simulink model "soc_WLAN_fpga"  (R2024b)
settings: Solver=FixedStepDiscrete  StartTime=0.0  StopTime=stopTime  RelTol=1e-3
PreLoadFcn:
  | addpath(fullfile(matlabroot,'toolbox','whdl','whdlexamples','whdlexamples'));
InitFcn:
  | addpath(fullfile(matlabroot,'toolbox','whdl','whdlexamples','whdlexamples'));
model workspace (MAT data in the model file):
  socvcb : containers.Map (value not decoded)
undefined symbols (not defined in the file): Add, bitRatePerOfdmSym, chanBW, coe, cpLen, dataUpsampleFactor, DelayValMaxNsdMinusLastPilotSc, DescramblerInitialSeed, designMultirateFIR, fftLen, filterLatency, filterUpsampleFactor, Fs, Hd, HT_MFMCS0, HT_MFMCS1, HT_MFMCS2, HT_MFMCS3, HT_MFMCS4, HT_MFMCS5, HT_MFMCS6, HT_MFMCS7, HTUnUsedScInd, inputSamplingRate, interp_coeff, maxPilotRefCounterVale, maxPilotsRef, maxPilotsRefNonHT, Ncol_HT, Ncol_NonHT, noDataSubCarriers, Non_HTMCS0, Non_HTMCS1, Non_HTMCS2, Non_HTMCS3, Non_HTMCS4, Non_HTMCS5, Non_HTMCS6, Non_HTMCS7, Nrow_HT, Nrow_NonHT, numDSC_HT, numDSC_HT_vhtSigB, numDSC_NonHT, numDscHT, numDscNonHT, numOfBitsPerOFDMSym, numOfDataBitsPerOFDMSym, numPilots, numScHT, numSCS_HT, numSCS_NonHT, pnSeq, QAM, rxDownsampleFactor, secondPIdx_HT, secondPIdx_NonHT, Shift, VHTMCS0, VHTMCS1 ... (+7)
libraries: hdlsllib x267, simulink x210, dspsigops x22, whdlutilities x10, whdlmod x9, dsphdlfiltering2 x5, dsphdlmathfun2 x4, whdledac x3, hwlogicconnlib x2, commhdlcrc x2, dsphdlsigops2 x2
(part 2 of 14)

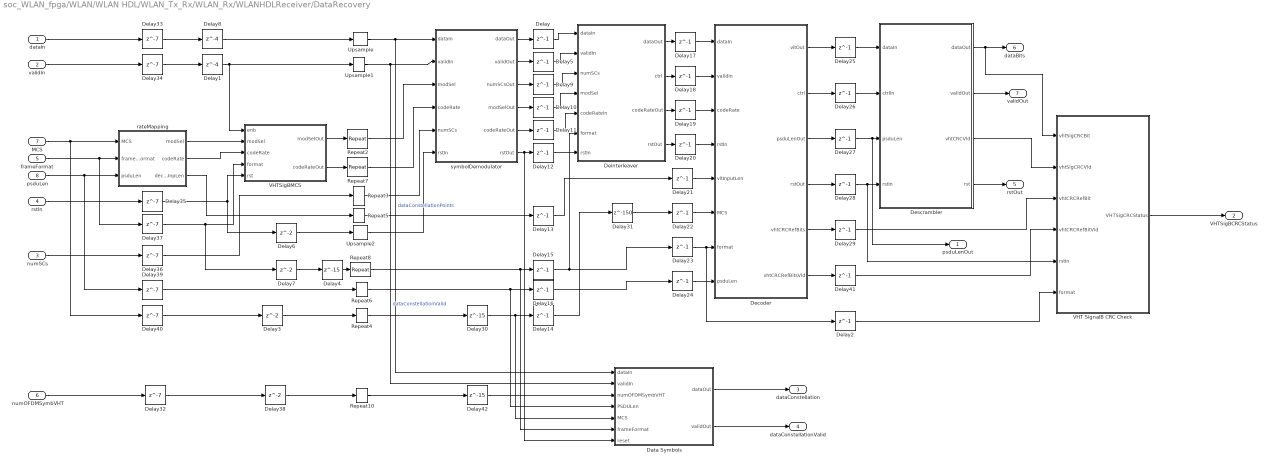
== system soc_WLAN_fpga/WLAN/WLAN HDL/WLAN_Tx_Rx/WLAN_Rx/WLANHDLReceiver/DataRecovery ==
  dataIn : Inport
  validIn : Inport  Port=2
  numSCs : Inport  Port=3
  rstIn : Inport  Port=4
  frameFormat : Inport  Port=5
  numOFDMSymbVHT : Inport  Port=6
  MCS : Inport  Port=7
  psduLen : Inport  Port=8
  Data Symbols : Subsystem
  Decoder : Subsystem
  Deinterleaver : Subsystem
  Delay{,2,5,9..29,41} (25 alike) : Delay  DelayLength=1
  Delay1 : Delay  DelayLength=4
  Delay{3,6..7,38} (4 alike) : Delay
  Delay30 : Delay  DelayLength=15
  Delay31 : Delay  DelayLength=150
  Delay{32..37,39..40} (8 alike) : Delay  DelayLength=7
  Delay4 : Delay  DelayLength=15
  Delay42 : Delay  DelayLength=15
  Delay8 : Delay  DelayLength=4
  Descrambler : Subsystem
  Repeat{2..8,10} (8 alike) : dspsigops/Repeat  FactorSource=Dialog parameter  N=dataUpsampleFactor  Nmax=16  RateOptions=Allow multirate processing  ic=0  mode=Unused parameter value
  Upsample : dspsigops/Upsample  FactorSource=Dialog parameter  N=dataUpsampleFactor  Nmax=16  phase=0  RateOptions=Allow multirate processing  ic=0  mode=Unused parameter value
  Upsample1 : dspsigops/Upsample  FactorSource=Dialog parameter  N=dataUpsampleFactor  Nmax=16  phase=0  RateOptions=Allow multirate processing  ic=0  mode=Unused parameter value
  Upsample2 : dspsigops/Upsample  FactorSource=Dialog parameter  N=dataUpsampleFactor  Nmax=16  phase=0  RateOptions=Allow multirate processing  ic=0  mode=Unused parameter value
  VHT SignalB CRC Check : Subsystem
  VHTSigBMCS : Subsystem
  rateMapping : Subsystem
  symbolDemodulator : Subsystem
  psduLenOut : Outport
  VHTSigBCRCStatus : Outport  Port=2
  dataConstellation : Outport  Port=3
  dataConstellationValid : Outport  Port=4
  rstOut : Outport  Port=5
  dataBits : Outport  Port=6
  validOut : Outport  Port=7
  wires:
  Descrambler/2(validOut) -> validOut/1
  Descrambler/1(dataOut) -> VHT SignalB CRC Check/1(vhtSigCRCBit), dataBits/1
  Upsample1/1 -> symbolDemodulator/2(validIn), Data Symbols/2(validIn)  "dataConstellationValid"
  Upsample/1 -> symbolDemodulator/1(dataIn), Data Symbols/1(dataIn)  "dataConstellationPoints"
  Delay28/1 -> VHT SignalB CRC Check/5(rstIn), Descrambler/4(rstIn)
  Delay26/1 -> Descrambler/2(ctrlIn)
  Delay25/1 -> Descrambler/1(dataIn)
  Delay24/1 -> Decoder/8(psduLen)
  Delay23/1 -> Delay2/1, Decoder/7(format)
  Delay22/1 -> Decoder/6(MCS)
  Delay21/1 -> Decoder/5(vitInputLen)
  Delay20/1 -> Decoder/4(rstIn)
  Delay19/1 -> Decoder/3(codeRate)
  Delay18/1 -> Decoder/2(validIn)
  Delay17/1 -> Decoder/1(dataIn)
  Delay16/1 -> Delay24/1
  Delay15/1 -> Deinterleaver/6(format), Delay23/1
  Delay14/1 -> Delay31/1
  Delay13/1 -> Delay21/1
  Delay12/1 -> Deinterleaver/7(rstIn)
  Delay11/1 -> Deinterleaver/5(codeRateIn)
  Delay10/1 -> Deinterleaver/4(modSel)
  Delay9/1 -> Deinterleaver/3(numSCs)
  Delay5/1 -> Deinterleaver/2(validIn)
  Delay/1 -> Deinterleaver/1(dataIn)
  Decoder/3(psduLenOut) -> Delay27/1
  Decoder/5(vhtCRCRefBits) -> Delay29/1
  symbolDemodulator/6(rstOut) -> Data Symbols/7(reset), Delay12/1
  rateMapping/3(decoderInpLen) -> Repeat5/1
  rateMapping/2(codeRate) -> VHTSigBMCS/3(codeRate)
  rateMapping/1(modSel) -> VHTSigBMCS/2(modSel)
  symbolDemodulator/5(codeRateOut) -> Delay11/1
  Deinterleaver/3(codeRateOut) -> Delay19/1
  Repeat7/1 -> symbolDemodulator/4(codeRate)
  VHTSigBMCS/1(modSelOut) -> Repeat2/1
  Delay7/1 -> Delay4/1
  frameFormat/1 -> Delay37/1, rateMapping/2(frameFormat)
  Delay6/1 -> Upsample2/1
  Decoder/4(rstOut) -> Delay28/1
  Deinterleaver/4(rstOut) -> Delay20/1
  Delay4/1 -> Repeat8/1
  Delay1/1 -> VHTSigBMCS/1(enb), Upsample1/1
  validIn/1 -> Delay34/1
  Delay8/1 -> Upsample/1
  Repeat4/1 -> Delay30/1
  MCS/1 -> Delay40/1, rateMapping/1(MCS)
  VHTSigBMCS/2(codeRateOut) -> Repeat7/1
  Repeat8/1 -> Data Symbols/6(frameFormat), Delay15/1
  Repeat6/1 -> Delay16/1, Data Symbols/4(PSDULen)
  Repeat5/1 -> Delay13/1
  Upsample2/1 -> symbolDemodulator/6(rstIn)
  Repeat3/1 -> symbolDemodulator/5(numSCs)
  Repeat2/1 -> symbolDemodulator/3(modSel)
  rstIn/1 -> Delay35/1
  symbolDemodulator/4(modSelOut) -> Delay10/1
  psduLen/1 -> Delay39/1, rateMapping/3(psduLen)
  Deinterleaver/2(ctrl) -> Delay18/1
  Deinterleaver/1(dataOut) -> Delay17/1
  Decoder/2(ctrl) -> Delay26/1
  Decoder/1(vitOut) -> Delay25/1
  numSCs/1 -> Delay36/1
  symbolDemodulator/2(validOut) -> Delay5/1
  symbolDemodulator/1(dataOut) -> Delay/1
  symbolDemodulator/3(numSCsOut) -> Delay9/1
  dataIn/1 -> Delay33/1
  Delay33/1 -> Delay8/1
  Delay34/1 -> Delay1/1
  Delay35/1 -> VHTSigBMCS/5(rst), Delay6/1
  Delay36/1 -> Repeat3/1
  Delay37/1 -> VHTSigBMCS/4(format), Delay7/1
  Delay39/1 -> Repeat6/1
  Delay40/1 -> Delay3/1
  Decoder/6(vhtCRCRefBitsVld) -> Delay41/1
  Descrambler/3(vhtCRCVld) -> VHT SignalB CRC Check/2(vhtSigCRCVld)
  Delay29/1 -> VHT SignalB CRC Check/3(vhtCRCRefBit)
  VHT SignalB CRC Check/1(VHTSigCRCStatus) -> VHTSigBCRCStatus/1
  Delay27/1 -> psduLenOut/1, Descrambler/3(psduLen)
  Data Symbols/2(validOut) -> dataConstellationValid/1
  Data Symbols/1(dataOut) -> dataConstellation/1
  Delay41/1 -> VHT SignalB CRC Check/4(vhtCRCRefBitVld)
  Delay2/1 -> VHT SignalB CRC Check/6(format)
  Delay3/1 -> Repeat4/1
  Delay30/1 -> Delay14/1, Data Symbols/5(MCS)
  Delay31/1 -> Delay22/1
  Delay32/1 -> Delay38/1
  Repeat10/1 -> Delay42/1
  Delay38/1 -> Repeat10/1
  numOFDMSymbVHT/1 -> Delay32/1
  Delay42/1 -> Data Symbols/3(numOFDMSymbVHT)
  Descrambler/4(rst) -> rstOut/1

== system soc_WLAN_fpga/WLAN/WLAN HDL/WLAN_Tx_Rx/WLAN_Rx/WLANHDLReceiver/FrameFormatController ==
  note: Appriopriate delays to match detected frame format arrival
  note: Choose L-Data from symbol 6
  NonHTDataIn : Inport
  NonHTValid : Inport  Port=2
  numSymb : Inport  Port=3
  NonHTRst : Inport  Port=4
  formatDetected : Inport  Port=5
  HTDataIn : Inport  Port=6
  HTValid : Inport  Port=7
  HTRst : Inport  Port=8
  Compare To Constant : simulink/Logic and Bit Operations/Compare To Constant  relop=>=  const=5  OutDataTypeStr=boolean
  Constant : Constant  Value=numDscHT  OutDataTypeStr=fixdt(0,16,0)  SampleTime=-1
  Constant1 : Constant  Value=numDscNonHT  OutDataTypeStr=fixdt(0,16,0)  SampleTime=-1
  Delay : Delay  DelayLength=388+64+160+64
  Delay10 : Delay  DelayLength=87+32+8*fftLen
  Delay11 : Delay  DelayLength=388+160+64+64
  Delay3 : Delay  DelayLength=87+32
  Delay4 : Delay  DelayLength=87+32
  Delay8 : Delay  DelayLength=388+64+160+64
  Delay9 : Delay  DelayLength=388+160+64+64
  Logical Operator : Logic  AllPortsSameDT=off  OutDataTypeStr=boolean
  Switch1 : Switch  Criteria=u2 > Threshold  SaturateOnIntegerOverflow=off  InputSameDT=off  OutDataTypeStr=Inherit: Same as first input
  Switch3 : Switch  Criteria=u2 > Threshold  SaturateOnIntegerOverflow=off  InputSameDT=off
  Switch4 : Switch  Criteria=u2 > Threshold  SaturateOnIntegerOverflow=off  InputSameDT=off
  Switch5 : Switch  Criteria=u2 > Threshold  SaturateOnIntegerOverflow=off  InputSameDT=off
  dataOut : Outport
  validOut : Outport  Port=2
  numSCs : Outport  Port=3
  rstOut : Outport  Port=4
  wires:
  Switch5/1 -> rstOut/1
  Switch1/1 -> dataOut/1
  Delay8/1 -> Logical Operator/1
  Constant/1 -> Switch4/1
  Compare To Constant/1 -> Logical Operator/2
  Constant1/1 -> Switch4/3
  Delay4/1 -> Switch1/1
  Delay/1 -> Compare To Constant/1
  Delay9/1 -> Switch1/3
  Switch4/1 -> numSCs/1
  Logical Operator/1 -> Switch3/3
  Delay3/1 -> Switch3/1
  Delay11/1 -> Switch5/3
  Delay10/1 -> Switch5/1
  numSymb/1 -> Delay/1
  HTRst/1 -> Delay10/1
  Switch3/1 -> validOut/1
  HTValid/1 -> Delay3/1
  HTDataIn/1 -> Delay4/1
  NonHTDataIn/1 -> Delay9/1
  NonHTValid/1 -> Delay8/1
  NonHTRst/1 -> Delay11/1
  formatDetected/1 -> Switch4/2, Switch5/2, Switch1/2, Switch3/2

== system soc_WLAN_fpga/WLAN/WLAN HDL/WLAN_Tx_Rx/WLAN_Rx/WLANHDLReceiver/FrameFormatDetectionAndSignalRecovery ==
  dataIn : Inport
  validIn : Inport  Port=2
  symbNum : Inport  Port=3
  rstIn : Inport  Port=4
  CRCCheckAndBitInterpretation : Subsystem
  Data Type Conversion : DataTypeConversion  OutDataTypeStr=fixdt(1,16,14)  SaturateOnIntegerOverflow=off  RndMeth=Floor
  Delay : Delay  DelayLength=18
  FormatIdentification : Subsystem
      settings: PortSchema="{\"entries\":[{\"content\":{\"sides\":[{\"content\":{\"connectorIds\":[\"In1\",\"In2\",\"In3\",\"In4\"]},\"type\":\"ConnectorPlacement.EquallySpacedRectSide\",\"uuid\":\"3028114e-cab1-417f-bebe-6d6476787930\"},{\"content\":{\"connectorIds\":[],\"side\":\"RIGHT\"},\"type\":\"ConnectorPlacement.EquallySpacedRectSide\",\"uuid\":\"6d8234fc-94fb-4772-a32f-944b1f5aeeb4\"},{\"content\":{\"connectorIds\":[\"Out2\",\"In5\"],\"side\":\"TOP\"},\"type\":\"ConnectorPlacement.EquallySpacedRectSide\",\"uuid\":\"0ff67b69-6efc-48c5-b813-d09036213c24\"},{\"content\":{\"connectorIds\":[\"Out1\"],\"side\":\"BOTTOM\"},\"type\":\"ConnectorPlacement.EquallySpacedRectSide\",\"uuid\":\"c34dfd74-148e-4ad2-9a51-cfec2f6e9138\"}]},\"type\":\"ConnectorPlacement.EquallySpacedConnector\",\"uuid\":\"49430930-ff4f-4485-8b33-823117f3dfd7\"}],\"packageUris\":[\"http://schema.mathworks.com/mf0/Connector/R2020b\"],\"version\":\"1.0\"}"
  Sample Control Bus Selector : whdlutilities/Sample Control Bus Selector  OutputSignals=start,end,valid
  SignalBitRecovery : Subsystem
  SignalFieldController : Subsystem
      settings: PortSchema="{\"entries\":[{\"content\":{\"sides\":[{\"content\":{\"connectorIds\":[\"In1\",\"In2\",\"In3\",\"In4\",\"In5\",\"In6\"]},\"type\":\"ConnectorPlacement.EquallySpacedRectSide\",\"uuid\":\"148ceb8f-1186-445b-b3f6-f8d5d753c1bf\"},{\"content\":{\"connectorIds\":[\"Out1\",\"Out2\",\"Out3\",\"Out4\"],\"side\":\"RIGHT\"},\"type\":\"ConnectorPlacement.EquallySpacedRectSide\",\"uuid\":\"6dacdfa0-ad7e-48bf-93e0-eecd8ec6f6a0\"},{\"content\":{\"connectorIds\":[],\"side\":\"TOP\"},\"type\":\"ConnectorPlacement.EquallySpacedRectSide\",\"uuid\":\"eaeaab77-8bbe-4397-bc6e-e6aaca64b8f0\"},{\"content\":{\"connectorIds\":[\"In7\"],\"side\":\"BOTTOM\"},\"type\":\"ConnectorPlacement.EquallySpacedRectSide\",\"uuid\":\"580f9177-349a-4b9d-9319-c70de4e7be3b\"}]},\"type\":\"ConnectorPlacement.EquallySpacedConnector\",\"uuid\":\"773ad17b-09fa-48bb-b0c0-63eaf23152dd\"}],\"packageUris\":[\"http://schema.mathworks.com/mf0/Connector/R2020b\"],\"version\":\"1.0\"}"
  Terminator10 : Terminator
  Terminator9 : Terminator
  averageSigFieldsFor40MHz : Subsystem
  storingSignalFields : Subsystem
      settings: PortSchema="{\"entries\":[{\"content\":{\"sides\":[{\"content\":{\"connectorIds\":[\"In1\",\"In2\",\"In3\",\"In4\"]},\"type\":\"ConnectorPlacement.EquallySpacedRectSide\",\"uuid\":\"994a7f9b-6ab5-43b4-a8d7-53561a33412d\"},{\"content\":{\"connectorIds\":[\"Out1\",\"Out2\"],\"side\":\"RIGHT\"},\"type\":\"ConnectorPlacement.EquallySpacedRectSide\",\"uuid\":\"f9668c3e-3593-48e7-8bc9-4614bf79b57c\"},{\"content\":{\"connectorIds\":[\"In5\"],\"side\":\"TOP\"},\"type\":\"ConnectorPlacement.EquallySpacedRectSide\",\"uuid\":\"29666b31-aec6-4c8c-a4b7-b4d610cf5f51\"}]},\"type\":\"ConnectorPlacement.EquallySpacedConnector\",\"uuid\":\"339975a6-4895-4382-8eec-20ecff8c26e4\"}],\"packageUris\":[\"http://schema.mathworks.com/mf0/Connector/R2020b\"],\"version\":\"1.0\"}"
  decodedMCS : Outport
  CRCCheck : Outport  Port=2
  frameFormat : Outport  Port=3
  PSDULength : Outport  Port=4
  HTCRCStatus : Outport  Port=5
  headerConstellation : Outport  Port=6
  numOFDMSymbVHT : Outport  Port=7
  wires:
  symbNum/1 -> FormatIdentification/3(symbCount), storingSignalFields/4(symbCount), SignalFieldController/5(symbNum)
  Sample Control Bus Selector/3 -> CRCCheckAndBitInterpretation/2(<valid>)  "<valid>"
  Sample Control Bus Selector/2 -> Terminator10/1  "<end>"
  SignalBitRecovery/2(ctrlOut) -> Sample Control Bus Selector/1
  Sample Control Bus Selector/1 -> Terminator9/1  "<start>"
  FormatIdentification/2(frameFormat) -> CRCCheckAndBitInterpretation/3(formatDetected), frameFormat/1, SignalFieldController/7(formatDetected)
  FormatIdentification/1(formatDetected) -> storingSignalFields/5(formatDetected)
  SignalFieldController/3(modSel) -> SignalBitRecovery/3(modSel)
  SignalFieldController/2(dataSCValid) -> SignalBitRecovery/2(dataSCValid)
  SignalFieldController/1(dataOut) -> SignalBitRecovery/1(dataIn)
  storingSignalFields/2(validOut) -> [HTSigSymbValid]
  [HTSigSymbValid] -> SignalFieldController/4(validOut)
  storingSignalFields/1(rd_dout) -> [HTSigSymbData]
  [HTSigSymbData] -> SignalFieldController/3(rd_dout)
  SignalBitRecovery/1(signBit) -> CRCCheckAndBitInterpretation/1(bit)
  rstIn/1 -> storingSignalFields/1(rst), FormatIdentification/4(rst), SignalFieldController/6(rst), SignalBitRecovery/4(rst), Delay/1, averageSigFieldsFor40MHz/3(rst)
  CRCCheckAndBitInterpretation/4(MCS) -> FormatIdentification/5(MCS), decodedMCS/1
  CRCCheckAndBitInterpretation/1(failCheck) -> CRCCheck/1
  CRCCheckAndBitInterpretation/2(PSDULen) -> PSDULength/1
  SignalBitRecovery/3(headerConstellation) -> headerConstellation/1
  CRCCheckAndBitInterpretation/3(HTCRCStatus) -> HTCRCStatus/1
  Data Type Conversion/1 -> storingSignalFields/2(dataIn), FormatIdentification/1(dataIn), SignalFieldController/1(dataIn)
  SignalFieldController/4(numSCS) -> SignalBitRecovery/5(numSCS)
  averageSigFieldsFor40MHz/2(Out2) -> SignalFieldController/2(validIn), storingSignalFields/3(validIn), FormatIdentification/2(validIn)
  dataIn/1 -> averageSigFieldsFor40MHz/1(In1)
  validIn/1 -> averageSigFieldsFor40MHz/2(In2)
  averageSigFieldsFor40MHz/1(Out1) -> Data Type Conversion/1
  Delay/1 -> CRCCheckAndBitInterpretation/4(rst)
  CRCCheckAndBitInterpretation/5(numOFDMSymbVHT) -> numOFDMSymbVHT/1

== system soc_WLAN_fpga/WLAN/WLAN HDL/WLAN_Tx_Rx/WLAN_Rx/WLANHDLReceiver/HT_VHTCPEEstAndCorrection ==
  dataIn : Inport
  validIn : Inport  Port=2
  vhtSigB : Inport  Port=3
  formatDetected : Inport  Port=4
  rstIn : Inport  Port=5
  CPECorrector : Subsystem
  CPEEstimator : Subsystem
  Data Type Conversion : DataTypeConversion  OutDataTypeStr=fixdt(1,16,10)  SaturateOnIntegerOverflow=off  RndMeth=Floor
  Data Type Conversion1 : DataTypeConversion  OutDataTypeStr=fixdt(1,16,14)  SaturateOnIntegerOverflow=off  RndMeth=Floor
  Delay{,1,3,9} (4 alike) : Delay
  Delay10 : Delay  DelayLength=3
  Delay11 : Delay  DelayLength=3
  Delay{12..23} (12 alike) : Delay  DelayLength=1  InitialCondition=0  UseCircularBuffer=on
  Delay2 : Delay  DelayLength=3
  Delay4 : Delay  DelayLength=fftLen
  Delay5 : Delay  DelayLength=fftLen
  Delay6 : Delay  DelayLength=fftLen
  Delay7 : Delay  DelayLength=1.5*(fftLen)
  Delay8 : Delay  DelayLength=94+56
  Logical Operator1 : Logic  AllPortsSameDT=off  OutDataTypeStr=boolean
  Logical Operator2 : Logic  Operator=NOT  AllPortsSameDT=off  OutDataTypeStr=boolean
  Logical Operator3 : Logic  Operator=OR  AllPortsSameDT=off  OutDataTypeStr=boolean
  PilotSubCarrierSelector : Subsystem
  PolarityGenerator : Subsystem
  dataOut : Outport
  validOut : Outport  Port=2
  rstOut : Outport  Port=3
  wires:
  Delay10/1 -> Data Type Conversion1/1
  Delay11/1 -> validOut/1
  Delay8/1 -> Delay2/1
  PilotSubCarrierSelector/3(SymbStart) -> PolarityGenerator/1(enb)
  PolarityGenerator/2(vhtSigB) -> CPEEstimator/5(vhtSigB)
  PilotSubCarrierSelector/2(SymbEndInd) -> Delay/1
  Logical Operator3/1 -> Delay16/1, PilotSubCarrierSelector/1(validIn)  "sampleIn"
  Delay/1 -> CPEEstimator/3(SymbolEndInd)
  Logical Operator2/1 -> Logical Operator1/2
  Delay9/1 -> Delay5/1
  Delay3/1 -> CPEEstimator/2(pilotScValid)
  Logical Operator1/1 -> Delay9/1  "sampleIn"
  Delay1/1 -> Data Type Conversion/1, CPEEstimator/1(dataOut)
  PolarityGenerator/1(polarity) -> CPEEstimator/4(polarity)
  PilotSubCarrierSelector/1(pilotScValidOut) -> Delay3/1, Logical Operator2/1  "sampleOut"
  CPECorrector/1(dataOut) -> Delay10/1
  validIn/1 -> Logical Operator3/1  "sampleIn"
  CPECorrector/2(validOut) -> Delay11/1
  Delay2/1 -> rstOut/1
  Data Type Conversion1/1 -> dataOut/1
  CPEEstimator/1(x) -> CPECorrector/3(estimate)
  formatDetected/1 -> Delay7/1
  Delay12/1 -> CPECorrector/1(dataIn)
  Delay13/1 -> CPECorrector/2(validIn)
  Delay14/1 -> Delay8/1
  Data Type Conversion/1 -> Delay4/1
  Delay6/1 -> Delay23/1
  Delay7/1 -> Delay17/1
  vhtSigB/1 -> Delay18/1, Logical Operator3/2
  dataIn/1 -> Delay15/1
  rstIn/1 -> Delay19/1, PilotSubCarrierSelector/2(rst)
  Delay5/1 -> Delay22/1
  Delay4/1 -> Delay21/1
  Delay15/1 -> Delay1/1
  Delay16/1 -> Logical Operator1/1
  Delay17/1 -> PolarityGenerator/2(formatDetected)
  Delay18/1 -> PolarityGenerator/3(VHTSigB)
  Delay19/1 -> Delay20/1, PolarityGenerator/4(rst)
  Delay20/1 -> Delay6/1, CPEEstimator/6(rst)
  Delay21/1 -> Delay12/1
  Delay22/1 -> Delay13/1
  Delay23/1 -> Delay14/1

== system soc_WLAN_fpga/WLAN/WLAN HDL/WLAN_Tx_Rx/WLAN_Rx/WLANHDLReceiver/HT_VHTChannelEstAndEqualize ==
  note: Delay by 1.4 times OFDM symbol length to match frame format detected
  note: HT/VHT scaling factor
  dataIn : Inport
  validIn : Inport  Port=2
  symbNum : Inport  Port=3
  symbRst : Inport  Port=4
  rstIn : Inport  Port=5
  formatIn : Inport  Port=6
  ChannelEqualizer : Subsystem
  ChannelEstimator : Subsystem
  Delay : Delay  DelayLength=80+32
  Delay15 : Delay  DelayLength=80+32
  Delay16 : Delay  DelayLength=80+32
  Delay{3..5,22..23} (5 alike) : Delay  DelayLength=14  InputProcessing=Columns as channels (frame based)
  Delay24 : Delay  DelayLength=94  InputProcessing=Columns as channels (frame based)
  Delay6 : Delay  DelayLength=94  InputProcessing=Columns as channels (frame based)
  Gain : Gain  Gain=fi(sqrt(numScHT),0,16,8)  OutDataTypeStr=fixdt(1,16,13)
  HTScSelector : Subsystem
  ValidController : Subsystem
  dataOut : Outport
  validOut : Outport  Port=2
  vhtSigBVld : Outport  Port=3
  formatOut : Outport  Port=4
  rstOut : Outport  Port=5
  wires:
  ChannelEstimator/3(chanEstLen) -> ChannelEqualizer/5(chanEstLen)
  Delay4/1 -> ChannelEqualizer/2(validIn)
  ChannelEstimator/1(HT_VHTchanEst) -> ChannelEqualizer/3(chanEst)
  HTScSelector/1(chanEstValid) -> Delay4/1, ChannelEstimator/2(validIn)
  Delay3/1 -> ChannelEqualizer/1(dataIn)
  Delay5/1 -> Delay6/1, ChannelEqualizer/7(symbNum)
  ChannelEstimator/2(HT_VHTchanEstValid) -> ChannelEqualizer/4(chanEstVal)
  ChannelEqualizer/2(validOut) -> Delay15/1  "sampleIn"
  ChannelEqualizer/1(dataOut) -> Delay16/1
  Delay6/1 -> Delay/1
  formatIn/1 -> ValidController/2(formatDetected), formatOut/1
  Delay/1 -> ValidController/1(symbNum)
  Delay15/1 -> ValidController/3(validIn)
  Delay22/1 -> ChannelEqualizer/6(syncStart)
  Delay23/1 -> Delay24/1
  dataIn/1 -> Gain/1
  ValidController/2(vhtSigB) -> vhtSigBVld/1
  Delay16/1 -> dataOut/1
  ValidController/1(validOut) -> validOut/1
  Delay24/1 -> rstOut/1
  validIn/1 -> HTScSelector/1(validIn)
  symbRst/1 -> HTScSelector/2(symbRst)
  Gain/1 -> ChannelEstimator/1(dataIn), Delay3/1
  rstIn/1 -> Delay23/1, Delay22/1, ChannelEstimator/3(syncStart), HTScSelector/3(rst)
  symbNum/1 -> Delay5/1, ChannelEstimator/4(symbNum)

== system soc_WLAN_fpga/WLAN/WLAN HDL/WLAN_Tx_Rx/WLAN_Rx/WLANHDLReceiver/NonHTCPEEstAndCorrection ==
  dataIn : Inport
  sampleIn : Inport  Port=2
  symbNum : Inport  Port=3
  rstIn : Inport  Port=4
  CPECorrector : Subsystem
  CPEEstimator : Subsystem
  DataSubCarrierSelector : Subsystem
  Delay{,3..4,7,9,11..25} (20 alike) : Delay  DelayLength=1  InitialCondition=0  UseCircularBuffer=on
  Delay1 : Delay  DelayLength=37
  Delay10 : Delay  DelayLength=fftLen
  Delay2 : Delay  DelayLength=37
  Delay5 : Delay  DelayLength=fftLen  InputProcessing=Columns as channels (frame based)
  Delay6 : Delay  DelayLength=fftLen  InputProcessing=Columns as channels (frame based)
  Delay8 : Delay  DelayLength=fftLen  InputProcessing=Columns as channels (frame based)
  PilotSubCarrierSelector : Subsystem
  PolarityGenerator : Subsystem
  dataOut : Outport
  validOut : Outport  Port=2
  symbNumOut : Outport  Port=3
  rstOut : Outport  Port=4
  wires:
  CPECorrector/2(validOut) -> validOut/1
  Delay8/1 -> Delay11/1
  CPECorrector/1(dataOut) -> dataOut/1
  Delay10/1 -> Delay9/1
  Delay5/1 -> Delay12/1
  PolarityGenerator/1(polarity) -> CPEEstimator/4(polarity)
  PilotSubCarrierSelector/3(SymbStart) -> PolarityGenerator/1(enb)
  CPEEstimator/1(x) -> CPECorrector/3(estimate)
  Delay6/1 -> Delay13/1
  DataSubCarrierSelector/1(dataScValidOut) -> Delay6/1  "sampleIn"
  PilotSubCarrierSelector/2(SymbEndInd) -> Delay17/1
  PilotSubCarrierSelector/1(pilotScValidOut) -> Delay16/1  "sampleOut"
  Delay1/1 -> rstOut/1
  Delay2/1 -> symbNumOut/1
  Delay/1 -> CPECorrector/1(dataIn)
  Delay3/1 -> CPECorrector/2(validIn)
  Delay4/1 -> Delay1/1
  Delay7/1 -> Delay2/1
  Delay9/1 -> Delay4/1
  Delay11/1 -> Delay7/1
  Delay12/1 -> Delay/1
  Delay13/1 -> Delay3/1
  Delay14/1 -> Delay8/1
  Delay15/1 -> CPEEstimator/5(rst), Delay10/1
  Delay16/1 -> CPEEstimator/2(pilotScValid)
  Delay17/1 -> CPEEstimator/3(SymbolEndInd)
  Delay18/1 -> CPEEstimator/1(dataOut)
  Delay20/1 -> Delay5/1
  sampleIn/1 -> Delay24/1, PilotSubCarrierSelector/1(EqValidIn)
  dataIn/1 -> Delay23/1, Delay25/1
  rstIn/1 -> Delay19/1, Delay22/1, PilotSubCarrierSelector/2(rst)
  symbNum/1 -> Delay21/1
  Delay19/1 -> Delay15/1
  Delay21/1 -> Delay14/1
  Delay22/1 -> DataSubCarrierSelector/2(rst), PolarityGenerator/2(rstIn)
  Delay23/1 -> Delay18/1
  Delay24/1 -> DataSubCarrierSelector/1(EqValidIn)
  Delay25/1 -> Delay20/1

== system soc_WLAN_fpga/WLAN/WLAN HDL/WLAN_Tx_Rx/WLAN_Rx/WLANHDLReceiver/NonHTChannelEstAndEqualize ==
  note: Non-HT scaling factor
  note: Select Non-HT frame format used subcarriers
  dataIn : Inport
  validIn : Inport  Port=2
  symbNum : Inport  Port=3
  symbRst : Inport  Port=4
  rstIn : Inport  Port=5
  ChannelEqualizer : Subsystem
  ChannelEstimator : Subsystem
  Delay{,1..2,8,14} (5 alike) : Delay
  Delay{10..13} (4 alike) : Delay  DelayLength=1
  Delay{3..5,7} (4 alike) : Delay  DelayLength=14  InputProcessing=Columns as channels (frame based)
  Delay6 : Delay  DelayLength=92  InputProcessing=Columns as channels (frame based)
  Delay9 : Delay  DelayLength=92  InputProcessing=Columns as channels (frame based)
  Gain : Gain  Gain=fi(sqrt(numSCS_NonHT),0,16,8)  OutDataTypeStr=fixdt(1,16,13)
  NonHTScSelector : Subsystem
  dataOut : Outport
  validOut : Outport  Port=2
  symbNumOut : Outport  Port=3
  rstOut : Outport  Port=4
  wires:
  Delay3/1 -> ChannelEqualizer/1(dataIn)
  Delay5/1 -> ChannelEqualizer/6(symbNum), Delay6/1
  Delay10/1 -> Delay3/1, ChannelEstimator/1(dataIn)
  Delay13/1 -> ChannelEstimator/4(syncStart), Delay7/1
  Delay9/1 -> rstOut/1
  Delay1/1 -> NonHTScSelector/1(validIn)
  Delay/1 -> Gain/1
  Delay11/1 -> ChannelEstimator/2(validIn), Delay4/1
  dataIn/1 -> Delay/1
  ChannelEstimator/2(chanEstValid) -> ChannelEqualizer/4(chanEstVal)
  Delay12/1 -> Delay5/1, ChannelEstimator/3(symbNum)
  ChannelEqualizer/2(validOut) -> validOut/1
  ChannelEqualizer/1(dataOut) -> dataOut/1
  symbNum/1 -> Delay2/1
  ChannelEstimator/3(chanEstLen) -> ChannelEqualizer/5(chanEstLen)
  rstIn/1 -> Delay8/1
  Delay6/1 -> symbNumOut/1
  Delay4/1 -> ChannelEqualizer/2(validIn)
  validIn/1 -> Delay1/1
  ChannelEstimator/1(chanEst) -> ChannelEqualizer/3(chanEst)
  NonHTScSelector/1(chanEstValid) -> Delay11/1
  Delay7/1 -> ChannelEqualizer/7(rst), Delay9/1
  symbRst/1 -> Delay14/1
  Delay14/1 -> NonHTScSelector/2(symbRst)
  Gain/1 -> Delay10/1
  Delay2/1 -> Delay12/1
  Delay8/1 -> Delay13/1, NonHTScSelector/3(rst)

== system soc_WLAN_fpga/WLAN/WLAN HDL/WLAN_Tx_Rx/WLAN_Rx/WLANHDLReceiver/OFDMDemodulation ==
  dataIn : Inport
  validIn : Inport  Port=2
  rstIn : Inport  Port=3
  Data Type Conversion : DataTypeConversion  OutDataTypeStr=fixdt(1,16,14)  SaturateOnIntegerOverflow=off  RndMeth=Floor
  Delay : Delay  DelayLength=278
  Delay{1..6} (6 alike) : Delay  DelayLength=1
  Delay7 : Delay
  Delay8 : Delay
  Delay9 : Delay
  Logical Operator : Logic  AllPortsSameDT=off  OutDataTypeStr=boolean
  Logical Operator1 : Logic  Operator=NOT  AllPortsSameDT=off  OutDataTypeStr=boolean
  OFDM Demodulator : whdlmod/OFDM Demodulator  OFDMParamsSource=Input port  MaxFFTLength=maxFFTLen  FFTLength=64  CPLength=16  NumLGsC=6  NumRGsC=5  CPFraction=off  CPFractionSource=Property  CPFractionValue=0.75  removeDCSubcarriers=off  enableResetInputPort=on  Normalize=on  RoundingMethod=Floor  SimulateUsing=Code generation
  OFDMDemodParamsCalculator : MATLAB Function  TreatAsAtomicUnit=on
  Symbol Counter : Subsystem
  Terminator4 : Terminator
  dataOut : Outport
  validOut : Outport  Port=2
  "symbNum " : Outport  Port=3
  symbRst : Outport  Port=4
  rstOut : Outport  Port=5
  wires:
  Delay7/1 -> Delay1/1
  Logical Operator/1 -> OFDM Demodulator/2
  Delay6/1 -> OFDM Demodulator/6
  OFDMDemodParamsCalculator/2(cpLen) -> Delay4/1
  OFDM Demodulator/2 -> Symbol Counter/1(validIn), validOut/1
  OFDMDemodParamsCalculator/1(fftLen) -> Delay3/1
  Logical Operator1/1 -> Logical Operator/2
  Delay2/1 -> Logical Operator/1
  Delay3/1 -> OFDM Demodulator/3
  OFDMDemodParamsCalculator/4(rgSc) -> Delay6/1
  OFDM Demodulator/3 -> Terminator4/1
  Delay/1 -> Symbol Counter/2(rst), rstOut/1
  OFDMDemodParamsCalculator/3(lgSc) -> Delay5/1
  Delay1/1 -> OFDM Demodulator/1
  Delay5/1 -> OFDM Demodulator/5
  Delay4/1 -> OFDM Demodulator/4
  dataIn/1 -> Delay7/1
  Delay9/1 -> Delay/1, OFDM Demodulator/7, OFDMDemodParamsCalculator/2(reset), Logical Operator1/1
  validIn/1 -> Delay8/1
  Symbol Counter/1(count) -> "symbNum "/1
  Data Type Conversion/1 -> dataOut/1
  Delay8/1 -> Delay2/1, OFDMDemodParamsCalculator/1(valid)
  rstIn/1 -> Delay9/1
  Symbol Counter/2(symbolRst) -> symbRst/1
  OFDM Demodulator/1 -> Symbol Counter/3(dataIn)
  Symbol Counter/3(dataOut) -> Data Type Conversion/1

== system soc_WLAN_fpga/WLAN/WLAN HDL/WLAN_Tx_Rx/WLAN_Rx/WLANHDLReceiver/WLANTimeAndFrequencySynchronization ==
  dataIn : Inport
  validIn : Inport  Port=2
  startIn : Inport  Port=3
  Add : Sum
  Coarse CFO Estimation and Correction : Subsystem
  Coarse Time Sync : Subsystem
  Data Type Conversion : DataTypeConversion  OutDataTypeStr=fixdt(1,14,14)  SaturateOnIntegerOverflow=off  RndMeth=Floor
  Delay : Delay  DelayLength=1
  Delay1 : Delay  DelayLength=1  InitialCondition=0
  Delay2 : Delay  DelayLength=1  InitialCondition=0
  Delay3 : Delay  DelayLength=1  InitialCondition=0
  Delay4 : Delay  DelayLength=1
  Delay5 : Delay  DelayLength=1
  Fine CFO Estimation and Correction : Subsystem
  Fine Time Sync : Subsystem
  Rx Filter : Subsystem
  Terminator2 : Terminator
  dataOut : Outport
  validOut : Outport  Port=2
  rstOut : Outport  Port=3
  freqOffset : Outport  Port=4
  wires:
  validIn/1 -> Delay2/1
  dataIn/1 -> Delay3/1
  startIn/1 -> Delay1/1
  Fine Time Sync/1(dataOut) -> Fine CFO Estimation and Correction/1(dataIn)
  Fine Time Sync/3(lstfStartOut) -> Fine CFO Estimation and Correction/3(lstfStartIn)
  Fine Time Sync/4(rstOut) -> Fine CFO Estimation and Correction/4(rstIn)
  Fine CFO Estimation and Correction/1(Freq) -> Add/2
  Add/1 -> Data Type Conversion/1
  Fine CFO Estimation and Correction/2(freqValidOut) -> Terminator2/1
  Coarse Time Sync/1(dataOut) -> Coarse CFO Estimation and Correction/1(dataIn)
  Data Type Conversion/1 -> freqOffset/1
  Fine Time Sync/2(validOut) -> Fine CFO Estimation and Correction/2(validIn)
  Delay3/1 -> Rx Filter/1(dataIn)
  Delay2/1 -> Rx Filter/2(validIn)
  Delay1/1 -> Rx Filter/3(startIn)
  Rx Filter/1(dataOut) -> Delay/1
  Rx Filter/2(validOut) -> Delay4/1
  Rx Filter/3(startOut) -> Delay5/1
  Delay/1 -> Coarse Time Sync/1(dataIn)
  Delay4/1 -> Coarse Time Sync/2(validIn)
  Delay5/1 -> Coarse Time Sync/3(startIn)
  Coarse Time Sync/3(lstfStart) -> Coarse CFO Estimation and Correction/3(lstfStartIn)
  Coarse Time Sync/4(rst) -> Coarse CFO Estimation and Correction/4(rstIn)
  Coarse CFO Estimation and Correction/1(Freq) -> Add/1
  Coarse CFO Estimation and Correction/4(lstfStartOut) -> Fine Time Sync/3(lstfStartIn)
  Coarse CFO Estimation and Correction/3(validOut) -> Fine Time Sync/2(validIn)
  Coarse CFO Estimation and Correction/5(rstOut) -> Fine Time Sync/4(rstIn)
  Coarse CFO Estimation and Correction/2(dataOut) -> Fine Time Sync/1(dataIn)
  Fine CFO Estimation and Correction/3(dataOut) -> dataOut/1
  Fine CFO Estimation and Correction/4(validOut) -> validOut/1
  Fine CFO Estimation and Correction/5(lstfStartOut) -> rstOut/1
  Coarse Time Sync/2(validOut) -> Coarse CFO Estimation and Correction/2(validIn)

== system soc_WLAN_fpga/WLAN/WLAN HDL/WLAN_Tx_Rx/WLAN_Rx/WLANHDLReceiver/diagBusControl ==
  MCS : Inport
  signalParity : Inport  Port=2
  frameFormatIn : Inport  Port=3
  HTSigCRCCheck : Inport  Port=4
  headerConst : Inport  Port=5
  packetOut : Inport  Port=6
  freqOff : Inport  Port=7
  psduLength : Inport  Port=8
  "VHTSigCRCCheck " : Inport  Port=9
  dataConst : Inport  Port=10
  dataConstValid : Inport  Port=11
  rst : Inport  Port=12
  Bus Creator : BusCreator  Inputs=2  OutDataTypeStr=Bus: dconstellationBus  NonVirtualBus=on
  Delay : Delay  DelayLength=1
  Enabled Delay{,1..3} (4 alike) : Delay  DelayLength=1  ShowEnablePort=on
      settings: InputPortMap=u0,e6
  Logical Operator : Logic  Operator=OR  AllPortsSameDT=off  OutDataTypeStr=boolean
  Logical Operator1 : Logic  Operator=OR  AllPortsSameDT=off  OutDataTypeStr=boolean
  Repeat{,1..2,4..5} (5 alike) : dspsigops/Repeat  FactorSource=Dialog parameter  N=8  Nmax=16  RateOptions=Allow multirate processing  ic=0  mode=Unused parameter value
  decodedMCS : Outport
  psduLen : Outport  Port=2
  signalParityStatus : Outport  Port=3
  signalCRCStatus : Outport  Port=4
  frameFormat : Outport  Port=5
  headerConstellation : Outport  Port=6
  dataConstellation : Outport  Port=7
  packetDetected : Outport  Port=8
  freqOffset : Outport  Port=9
  wires:
  rst/1 -> Delay/1, Logical Operator1/1
  Enabled Delay1/1 -> decodedMCS/1  "decodedMCS"
  Enabled Delay2/1 -> frameFormat/1  "frameFormat"
  signalParity/1 -> Repeat1/1
  Repeat4/1 -> packetDetected/1  "packetDetected"
  packetOut/1 -> Repeat4/1
  freqOff/1 -> Repeat5/1
  HTSigCRCCheck/1 -> Logical Operator/1
  "VHTSigCRCCheck "/1 -> Logical Operator/2
  Enabled Delay/1 -> psduLen/1
  Delay/1 -> Logical Operator1/2
  Repeat/1 -> Enabled Delay1/1  "decodedMCS"
  Repeat2/1 -> Enabled Delay2/1  "frameFormat"
  Repeat1/1 -> signalParityStatus/1  "signalPerity"
  psduLength/1 -> Enabled Delay/1
  MCS/1 -> Repeat/1
  frameFormatIn/1 -> Repeat2/1
  Bus Creator/1 -> dataConstellation/1
  Logical Operator/1 -> signalCRCStatus/1
  Logical Operator1/1 -> Enabled Delay2/2, Enabled Delay1/2, Enabled Delay3/2, Enabled Delay/2
  dataConst/1 -> Bus Creator/1  "dataConstellationPoints"
  dataConstValid/1 -> Bus Creator/2  "dataConstellationValid"
  headerConst/1 -> headerConstellation/1
  Repeat5/1 -> Enabled Delay3/1
  Enabled Delay3/1 -> freqOffset/1  "freqOffset"

== system soc_WLAN_fpga/WLAN/WLAN HDL/WLAN_Tx_Rx/WLAN_Tx/WLAN_Tx_20MHz/Tx_LUT_Selection ==
  note: Inputs are sampled only when counter reach zero
  LUTSelect : Inport
  Compare To Constant : simulink/Logic and Bit Operations/Compare To Constant  relop===  const=0  OutDataTypeStr=boolean
  Delay : Delay  DelayLength=1
  Frame Format 0 : Subsystem
      settings: PortSchema="{\"entries\":[{\"content\":{\"sides\":[{\"content\":{\"connectorIds\":[\"In1\",\"Out9\"]},\"type\":\"ConnectorPlacement.EquallySpacedRectSide\",\"uuid\":\"90f4e6e7-c75d-47eb-b46f-c1dc70fa163f\"},{\"content\":{\"connectorIds\":[\"Out1\",\"Out2\",\"Out3\",\"Out4\",\"Out5\",\"Out6\",\"Out7\",\"Out8\"],\"side\":\"RIGHT\"},\"type\":\"ConnectorPlacement.EquallySpacedRectSide\",\"uuid\":\"00a7ad00-c9d8-4450-becb-c58eec732ee4\"},{\"content\":{\"side\":\"TOP\"},\"type\":\"ConnectorPlacement.EquallySpacedRectSide\",\"uuid\":\"debcc5d2-c7ae-4348-934f-c91e3c4bc561\"}]},\"type\":\"ConnectorPlacement.EquallySpacedConnector\",\"uuid\":\"38ed2989-9419-4049-b4ae-20b01aa0fe2f\"}],\"packageUris\":[\"http://schema.mathworks.com/mf0/Connector/R2020b\"],\"version\":\"1.0\"}"
  Frame Format 1 : Subsystem
      settings: PortSchema="{\"entries\":[{\"content\":{\"sides\":[{\"content\":{\"connectorIds\":[\"In1\",\"Out9\"]},\"type\":\"ConnectorPlacement.EquallySpacedRectSide\",\"uuid\":\"90f4e6e7-c75d-47eb-b46f-c1dc70fa163f\"},{\"content\":{\"connectorIds\":[\"Out1\",\"Out2\",\"Out3\",\"Out4\",\"Out5\",\"Out6\",\"Out7\",\"Out8\"],\"side\":\"RIGHT\"},\"type\":\"ConnectorPlacement.EquallySpacedRectSide\",\"uuid\":\"00a7ad00-c9d8-4450-becb-c58eec732ee4\"},{\"content\":{\"side\":\"TOP\"},\"type\":\"ConnectorPlacement.EquallySpacedRectSide\",\"uuid\":\"debcc5d2-c7ae-4348-934f-c91e3c4bc561\"}]},\"type\":\"ConnectorPlacement.EquallySpacedConnector\",\"uuid\":\"38ed2989-9419-4049-b4ae-20b01aa0fe2f\"}],\"packageUris\":[\"http://schema.mathworks.com/mf0/Connector/R2020b\"],\"version\":\"1.0\"}"
  Frame Format 2 : Subsystem
      settings: PortSchema="{\"entries\":[{\"content\":{\"sides\":[{\"content\":{\"connectorIds\":[\"In1\",\"Out9\"]},\"type\":\"ConnectorPlacement.EquallySpacedRectSide\",\"uuid\":\"90f4e6e7-c75d-47eb-b46f-c1dc70fa163f\"},{\"content\":{\"connectorIds\":[\"Out1\",\"Out2\",\"Out3\",\"Out4\",\"Out5\",\"Out6\",\"Out7\",\"Out8\"],\"side\":\"RIGHT\"},\"type\":\"ConnectorPlacement.EquallySpacedRectSide\",\"uuid\":\"00a7ad00-c9d8-4450-becb-c58eec732ee4\"},{\"content\":{\"side\":\"TOP\"},\"type\":\"ConnectorPlacement.EquallySpacedRectSide\",\"uuid\":\"debcc5d2-c7ae-4348-934f-c91e3c4bc561\"}]},\"type\":\"ConnectorPlacement.EquallySpacedConnector\",\"uuid\":\"38ed2989-9419-4049-b4ae-20b01aa0fe2f\"}],\"packageUris\":[\"http://schema.mathworks.com/mf0/Connector/R2020b\"],\"version\":\"1.0\"}"
  HDL Counter : hdlsllib/Sources/HDL Counter  CountType=Count limited  CountInit=0  CountStep=1  CountMax=12479  CountFromType=Initial value  CountFrom=0  CountResetPort=on  CountLoadPort=off  CountEnbPort=off  CountDirPort=off  CountHitOutputPort=off  CountDataType=Unsigned  CountWordLen=16  CountFracLen=0  CountSampTime=1/(wlanConfig.Fs*2)
  Multiport Switch : MultiPortSwitch  DataPortOrder=Zero-based contiguous  Inputs=24  DiagnosticForDefault=Warning  zeroidx=on  SaturateOnIntegerOverflow=off  InputSameDT=off
  OR : Logic  Operator=OR  Inputs=3  IconShape=distinctive  AllPortsSameDT=off  OutDataTypeStr=boolean
  Unit Delay Enabled Synchronous : hdlsllib/Discrete/Unit Delay Enabled Synchronous  InitialCondition=0.0  SampleTime=-1
  txData : Outport
  wires:
  Multiport Switch/1 -> txData/1
  LUTSelect/1 -> Unit Delay Enabled Synchronous/1
  HDL Counter/1 -> Compare To Constant/1
  Compare To Constant/1 -> Unit Delay Enabled Synchronous/2
  Unit Delay Enabled Synchronous/1 -> Delay/1, Frame Format 2/1(enb), Frame Format 1/1(enb), Frame Format 0/1(enb)
  Frame Format 0/1(Outport) -> Multiport Switch/2
  Frame Format 0/2(Outport1) -> Multiport Switch/3
  Frame Format 0/3(Outport2) -> Multiport Switch/4
  Frame Format 0/4(Outport3) -> Multiport Switch/5
  Frame Format 0/5(Outport4) -> Multiport Switch/6
  Frame Format 0/6(Outport5) -> Multiport Switch/7
  Frame Format 0/7(Outport6) -> Multiport Switch/8
  Frame Format 0/8(Outport7) -> Multiport Switch/9
  Frame Format 1/1(Outport) -> Multiport Switch/10
  Frame Format 1/2(Outport1) -> Multiport Switch/11
  Frame Format 1/3(Outport2) -> Multiport Switch/12
  Frame Format 1/4(Outport3) -> Multiport Switch/13
  Frame Format 1/5(Outport4) -> Multiport Switch/14
  Frame Format 1/6(Outport5) -> Multiport Switch/15
  Frame Format 1/7(Outport6) -> Multiport Switch/16
  Frame Format 1/8(Outport7) -> Multiport Switch/17
  Frame Format 2/1(Outport) -> Multiport Switch/18
  Frame Format 2/2(Outport1) -> Multiport Switch/19
  Frame Format 2/3(Outport2) -> Multiport Switch/20
  Frame Format 2/4(Outport3) -> Multiport Switch/21
  Frame Format 2/5(Outport4) -> Multiport Switch/22
  Frame Format 2/6(Outport5) -> Multiport Switch/23
  Frame Format 2/7(Outport6) -> Multiport Switch/24
  Frame Format 2/8(Outport7) -> Multiport Switch/25
  Delay/1 -> Multiport Switch/1
  Frame Format 0/9(resetOut) -> OR/1
  Frame Format 1/9(resetOut) -> OR/2
  OR/1 -> HDL Counter/1
  Frame Format 2/9(resetOut) -> OR/3

== system soc_WLAN_fpga/WLAN/WLAN HDL/WLAN_Tx_Rx/WLAN_Tx/WLAN_Tx_40MHz/Tx_LUT_Selection ==
  note: Inputs are sampled only when counter reach zero
  LUTSelect : Inport
  Compare To Constant : simulink/Logic and Bit Operations/Compare To Constant  relop===  const=0  OutDataTypeStr=boolean
  Delay : Delay  DelayLength=1
  Frame Format 1 : Subsystem
      settings: PortSchema="{\"entries\":[{\"content\":{\"sides\":[{\"content\":{\"connectorIds\":[\"In1\",\"Out9\"]},\"type\":\"ConnectorPlacement.EquallySpacedRectSide\",\"uuid\":\"90f4e6e7-c75d-47eb-b46f-c1dc70fa163f\"},{\"content\":{\"connectorIds\":[\"Out1\",\"Out2\",\"Out3\",\"Out4\",\"Out5\",\"Out6\",\"Out7\",\"Out8\"],\"side\":\"RIGHT\"},\"type\":\"ConnectorPlacement.EquallySpacedRectSide\",\"uuid\":\"00a7ad00-c9d8-4450-becb-c58eec732ee4\"},{\"content\":{\"side\":\"TOP\"},\"type\":\"ConnectorPlacement.EquallySpacedRectSide\",\"uuid\":\"debcc5d2-c7ae-4348-934f-c91e3c4bc561\"}]},\"type\":\"ConnectorPlacement.EquallySpacedConnector\",\"uuid\":\"38ed2989-9419-4049-b4ae-20b01aa0fe2f\"}],\"packageUris\":[\"http://schema.mathworks.com/mf0/Connector/R2020b\"],\"version\":\"1.0\"}"
  Frame Format 2 : Subsystem
      settings: PortSchema="{\"entries\":[{\"content\":{\"sides\":[{\"content\":{\"connectorIds\":[\"In1\",\"Out9\"]},\"type\":\"ConnectorPlacement.EquallySpacedRectSide\",\"uuid\":\"90f4e6e7-c75d-47eb-b46f-c1dc70fa163f\"},{\"content\":{\"connectorIds\":[\"Out1\",\"Out2\",\"Out3\",\"Out4\",\"Out5\",\"Out6\",\"Out7\",\"Out8\"],\"side\":\"RIGHT\"},\"type\":\"ConnectorPlacement.EquallySpacedRectSide\",\"uuid\":\"00a7ad00-c9d8-4450-becb-c58eec732ee4\"},{\"content\":{\"side\":\"TOP\"},\"type\":\"ConnectorPlacement.EquallySpacedRectSide\",\"uuid\":\"debcc5d2-c7ae-4348-934f-c91e3c4bc561\"}]},\"type\":\"ConnectorPlacement.EquallySpacedConnector\",\"uuid\":\"38ed2989-9419-4049-b4ae-20b01aa0fe2f\"}],\"packageUris\":[\"http://schema.mathworks.com/mf0/Connector/R2020b\"],\"version\":\"1.0\"}"
  HDL Counter : hdlsllib/Sources/HDL Counter  CountType=Count limited  CountInit=0  CountStep=1  CountMax=7400  CountFromType=Initial value  CountFrom=0  CountResetPort=on  CountLoadPort=off  CountEnbPort=off  CountDirPort=off  CountHitOutputPort=off  CountDataType=Unsigned  CountWordLen=16  CountFracLen=0  CountSampTime=1/(wlanConfig.Fs*2)
  Multiport Switch : MultiPortSwitch  DataPortOrder=Zero-based contiguous  Inputs=16  DiagnosticForDefault=Warning  zeroidx=on  SaturateOnIntegerOverflow=off  InputSameDT=off
  OR : Logic  Operator=OR  IconShape=distinctive  AllPortsSameDT=off  OutDataTypeStr=boolean
  Unit Delay Enabled Synchronous : hdlsllib/Discrete/Unit Delay Enabled Synchronous  InitialCondition=0.0  SampleTime=-1
  txData : Outport
  wires:
  Multiport Switch/1 -> txData/1
  LUTSelect/1 -> Unit Delay Enabled Synchronous/1
  HDL Counter/1 -> Compare To Constant/1
  Compare To Constant/1 -> Unit Delay Enabled Synchronous/2
  Unit Delay Enabled Synchronous/1 -> Delay/1, Frame Format 2/1(enb), Frame Format 1/1(enb)
  Frame Format 1/1(Outport) -> Multiport Switch/2
  Frame Format 1/2(Outport1) -> Multiport Switch/3
  Frame Format 1/3(Outport2) -> Multiport Switch/4
  Frame Format 1/4(Outport3) -> Multiport Switch/5
  Frame Format 1/5(Outport4) -> Multiport Switch/6
  Frame Format 1/6(Outport5) -> Multiport Switch/7
  Frame Format 1/7(Outport6) -> Multiport Switch/8
  Frame Format 1/8(Outport7) -> Multiport Switch/9
  Frame Format 2/1(Outport) -> Multiport Switch/10
  Frame Format 2/2(Outport1) -> Multiport Switch/11
  Frame Format 2/3(Outport2) -> Multiport Switch/12
  Frame Format 2/4(Outport3) -> Multiport Switch/13
  Frame Format 2/5(Outport4) -> Multiport Switch/14
  Frame Format 2/6(Outport5) -> Multiport Switch/15
  Frame Format 2/7(Outport6) -> Multiport Switch/16
  Frame Format 2/8(Outport7) -> Multiport Switch/17
  Delay/1 -> Multiport Switch/1
  Frame Format 1/9(resetOut) -> OR/1
  Frame Format 2/9(resetOut) -> OR/2
  OR/1 -> HDL Counter/1

== system soc_WLAN_fpga/WLAN/WLAN HDL/WLAN_Tx_Rx/WLAN_Rx/WLANHDLReceiver/DataRecovery/Data Symbols ==
  dataIn : Inport
  validIn : Inport  Port=2
  numOFDMSymbVHT : Inport  Port=3
  PSDULen : Inport  Port=4
  MCS : Inport  Port=5
  frameFormat : Inport  Port=6
  reset : Inport  Port=7
  1-D Lookup Table2 : Lookup_n-D  NumberOfTableDimensions=1  BreakpointsForDimension1=[0:7]  IndexSearchMethod=Evenly spaced points  Table=bitRatePerOfdmSym*numDSC_HT  TableDataTypeStr=fixdt(1,16,13)  ExtrapMethod=Clip  UseLastTableValue=on  InternalRulePriority=Speed  OutDataTypeStr=fixdt(1,16,13)  RndMeth=Simplest
  AND1 : Logic  Inputs=3  AllPortsSameDT=off  OutDataTypeStr=boolean
  AND2 : Logic  AllPortsSameDT=off  OutDataTypeStr=boolean
  Compare To Constant1 : simulink/Logic and Bit Operations/Compare To Constant  relop===  const=2  OutDataTypeStr=boolean
  Compare To Constant2 : simulink/Logic and Bit Operations/Compare To Constant  relop=<  const=numDSC_HT  OutDataTypeStr=boolean
  Constant : Constant  Value=numDSC_HT  OutDataTypeStr=uint8  SampleTime=-1
  Data Type Conversion : DataTypeConversion  OutDataTypeStr=uint16  SaturateOnIntegerOverflow=off  RndMeth=Floor
  Delay{9..10,12,14} (4 alike) : Delay
  Delay11 : Delay  DelayLength=1
  Delay13 : Delay  DelayLength=1
  Delay6 : Delay  DelayLength=8
  Delay7 : Delay  DelayLength=8
  HDL Counter : hdlsllib/Sources/HDL Counter  CountType=Count limited  CountInit=0  CountStep=1  CountMax=65535  CountFromType=Initial value  CountFrom=0  CountResetPort=on  CountLoadPort=off  CountEnbPort=on  CountDirPort=off  CountHitOutputPort=off  CountDataType=Unsigned  CountWordLen=16  CountFracLen=0  CountSampTime=1
  NOT : Logic  Operator=NOT  AllPortsSameDT=off  OutDataTypeStr=boolean
  Product : Product  OutDataTypeStr=uint16
  Product5 : Product  RndMeth=Ceiling
  Relational Operator : RelationalOperator  Operator=<  OutDataTypeStr=boolean  RndMeth=Simplest  InputSameDT=off
  Shift Arithmetic : ArithShift  BitShiftNumber=3  BitShiftDirection=Left
  Switch1 : Switch  Threshold=2  SaturateOnIntegerOverflow=off  InputSameDT=off
  dataOut : Outport
  validOut : Outport  Port=2
  wires:
  Delay6/1 -> dataOut/1
  Delay7/1 -> validOut/1
  frameFormat/1 -> Switch1/2, Compare To Constant1/1
  Compare To Constant1/1 -> AND2/2
  numOFDMSymbVHT/1 -> Delay9/1
  Constant/1 -> Delay10/1
  validIn/1 -> HDL Counter/2, AND1/1
  HDL Counter/1 -> Compare To Constant2/1, Relational Operator/1
  Product/1 -> Delay11/1
  Relational Operator/1 -> AND1/2
  AND1/1 -> Delay7/1
  dataIn/1 -> Delay6/1
  reset/1 -> HDL Counter/1
  Delay9/1 -> Product/1
  Delay10/1 -> Product/2
  Compare To Constant2/1 -> AND2/1
  AND2/1 -> NOT/1
  NOT/1 -> AND1/3
  Product5/1 -> Data Type Conversion/1
  Delay14/1 -> Product5/2
  Shift Arithmetic/1 -> Delay12/1
  Delay12/1 -> Product5/1
  1-D Lookup Table2/1 -> Delay14/1
  PSDULen/1 -> Shift Arithmetic/1
  MCS/1 -> 1-D Lookup Table2/1
  Delay11/1 -> Switch1/1
  Delay13/1 -> Switch1/3
  Switch1/1 -> Relational Operator/2
  Data Type Conversion/1 -> Delay13/1

== system soc_WLAN_fpga/WLAN/WLAN HDL/WLAN_Tx_Rx/WLAN_Rx/WLANHDLReceiver/DataRecovery/Decoder ==
  dataIn : Inport
  validIn : Inport  Port=2
  codeRate : Inport  Port=3
  rstIn : Inport  Port=4
  vitInputLen : Inport  Port=5
  MCS : Inport  Port=6
  format : Inport  Port=7
  psduLen : Inport  Port=8
  Data Type Conversion : DataTypeConversion  OutDataTypeStr=uint16  SaturateOnIntegerOverflow=off  RndMeth=Floor
  Delay : Delay  DelayLength=1  InitialCondition=1000
  Delay1 : Delay  DelayLength=1  InitialCondition=1000
  Delay2 : Delay  DelayLength=5
  Delay3 : Delay  DelayLength=300
  Delay4 : Delay  DelayLength=10
  Delay5 : Delay  DelayLength=10
  Depuncturer : Subsystem
  Switch : Switch  Criteria=u2 > Threshold  Threshold=1  SaturateOnIntegerOverflow=off  InputSameDT=off
  Switch1 : Switch  Criteria=u2 > Threshold  Threshold=1  SaturateOnIntegerOverflow=off  InputSameDT=off
  ViterbiDecoder : Subsystem
  vhtSigB : Subsystem
  vitOut : Outport
  ctrl : Outport  Port=2
  psduLenOut : Outport  Port=3
  rstOut : Outport  Port=4
  vhtCRCRefBits : Outport  Port=5
  vhtCRCRefBitsVld : Outport  Port=6
  wires:
  Delay/1 -> Switch/1
  Switch/1 -> Depuncturer/4(vitInputLen)
  vitInputLen/1 -> Switch/3
  format/1 -> Depuncturer/5(format), vhtSigB/5(format), Switch1/2, Switch/2
  psduLen/1 -> Switch1/3
  Delay1/1 -> Switch1/1
  Switch1/1 -> Data Type Conversion/1
  dataIn/1 -> Depuncturer/1(dataIn)
  validIn/1 -> Depuncturer/2(ctrlIn)
  codeRate/1 -> Depuncturer/3(codeRate)
  rstIn/1 -> Depuncturer/6(rstIn), Delay2/1
  Delay2/1 -> Delay3/1
  Delay3/1 -> Delay4/1, vhtSigB/2(rst)
  ViterbiDecoder/1(bit) -> vhtSigB/3(bit), Delay5/1
  Depuncturer/1(dataOut) -> ViterbiDecoder/1(llr)
  Depuncturer/2(ctrl) -> ViterbiDecoder/2(validIn)
  MCS/1 -> vhtSigB/1(MCS)
  ViterbiDecoder/2(validOut) -> vhtSigB/4(ctrlIn)
  vhtSigB/1(ctrlOut) -> ctrl/1
  vhtSigB/2(vitInputLen) -> Delay/1
  vhtSigB/3(psduLen) -> Delay1/1
  Delay4/1 -> rstOut/1
  Delay5/1 -> vitOut/1
  Data Type Conversion/1 -> psduLenOut/1
  vhtSigB/4(vhtCRCRefBits) -> vhtCRCRefBits/1
  vhtSigB/5(vhtCRCRefBitsVld) -> vhtCRCRefBitsVld/1

== system soc_WLAN_fpga/WLAN/WLAN HDL/WLAN_Tx_Rx/WLAN_Rx/WLANHDLReceiver/DataRecovery/Deinterleaver ==
  note: Accumulated delay for reset to match both Deinterleaver outputs
  note: choose output based on block size
  note: Deinterleaver for Non-HT frame with block size 48
  note: Deinterleaver for HT/VHT frame with block size 52
  dataIn : Inport
  validIn : Inport  Port=2
  numSCs : Inport  Port=3
  modSel : Inport  Port=4
  codeRateIn : Inport  Port=5
  format : Inport  Port=6
  rstIn : Inport  Port=7
  Compare To Constant1 : simulink/Logic and Bit Operations/Compare To Constant  relop===  const=numSCS_NonHT-numPilots-1  OutDataTypeStr=boolean
  DeInterleaver_HT : Subsystem
  DeInterleaver_NonHT : Subsystem
  Delay : Delay  DelayLength=423
  Delay1 : Delay  DelayLength=1
  Delay2 : Delay  DelayLength=1
  Delay3 : Delay  DelayLength=52
  Sample Control Bus Creator : whdlutilities/Sample Control Bus Creator
  Sample Control Bus Creator1 : whdlutilities/Sample Control Bus Creator
  Switch1 : Switch  Criteria=u2 > Threshold  SaturateOnIntegerOverflow=off  InputSameDT=off
  Switch2 : Switch  Criteria=u2 > Threshold  SaturateOnIntegerOverflow=off  InputSameDT=off
  Terminator : Terminator
  Terminator3 : Terminator
  averageVhtSigBbits : Subsystem
  mapmodSelTobps : MATLAB Function  TreatAsAtomicUnit=on
  dataOut : Outport
  ctrl : Outport  Port=2
  codeRateOut : Outport  Port=3
  rstOut : Outport  Port=4
  wires:
  DeInterleaver_HT/3(endOut) -> averageVhtSigBbits/3(endIn)
  DeInterleaver_HT/6(ready) -> Terminator3/1
  DeInterleaver_NonHT/5(ready) -> Terminator/1
  DeInterleaver_HT/2(startOut) -> averageVhtSigBbits/2(startIn)
  validIn/1 -> DeInterleaver_NonHT/2(enb), DeInterleaver_HT/2(enb)
  dataIn/1 -> DeInterleaver_HT/1(wr_din), DeInterleaver_NonHT/1(wr_din)
  Compare To Constant1/1 -> Switch1/2, Switch2/2
  Switch2/1 -> ctrl/1
  numSCs/1 -> DeInterleaver_HT/5(numSCs), DeInterleaver_NonHT/5(numSCs), Compare To Constant1/1
  modSel/1 -> mapmodSelTobps/1(modSel)
  mapmodSelTobps/1(bps) -> DeInterleaver_NonHT/3(bps), DeInterleaver_HT/3(bps)
  rstIn/1 -> Delay2/1, DeInterleaver_HT/4(rstIn), averageVhtSigBbits/7(rst), DeInterleaver_NonHT/4(rst)
  Sample Control Bus Creator1/1 -> Switch2/1
  Sample Control Bus Creator/1 -> Switch2/3
  DeInterleaver_HT/4(validOut) -> averageVhtSigBbits/4(validIn)
  Delay/1 -> rstOut/1
  codeRateIn/1 -> Delay1/1
  Switch1/1 -> dataOut/1
  Delay2/1 -> Delay/1
  Delay1/1 -> Delay3/1
  DeInterleaver_NonHT/1(dataOut) -> Switch1/1
  DeInterleaver_NonHT/2(startOut) -> Sample Control Bus Creator1/1
  DeInterleaver_NonHT/3(endOut) -> Sample Control Bus Creator1/2
  DeInterleaver_NonHT/4(validOut) -> Sample Control Bus Creator1/3
  DeInterleaver_HT/1(dataOut) -> averageVhtSigBbits/1(dataIn)
  averageVhtSigBbits/1(dataOut) -> Switch1/3
  averageVhtSigBbits/3(endOut) -> Sample Control Bus Creator/2
  averageVhtSigBbits/2(startOut) -> Sample Control Bus Creator/1
  averageVhtSigBbits/4(validOut) -> Sample Control Bus Creator/3
  DeInterleaver_HT/5(numSCSFlag) -> averageVhtSigBbits/5(numSCSFlag)
  format/1 -> averageVhtSigBbits/6(format)
  Delay3/1 -> codeRateOut/1
